simulink model "ulise_internal_v0"  (R2025b)
settings: Solver=FixedStepDiscrete  StartTime=0.0  StopTime=999  FixedStep=1  RelTol=1e-3
model workspace (MAT data in the model file):
  Something = 3
values from neighbouring files (symbols this model uses):
  A = [0.5    2   0   0   0 ... (first row only)    [simulink_ULISE.m]
  B = zeros(size(A,1),1)    [simulink_ULISE.m]
  C = blkdiag(1,1,1,1,1)    [simulink_ULISE.m]
  D = zeros(size(C,1),1)    [simulink_ULISE.m]
  G = [1  0   -0.3 ... (first row only)    [simulink_ULISE.m]
  H = [0  0   1 ... (first row only)    [simulink_ULISE.m]
  K = 1000    [simulink_ULISE.m]
  Q = 1e-4* [1    0   0   0   0 ... (first row only)    [simulink_ULISE.m]
  R = 1e-2* [1    0   0   0.5 0 ... (first row only)    [simulink_ULISE.m]
  x = zeros(size(A,1),K)    [simulink_ULISE.m]
  x0 = zeros(size(A,1),1)    [simulink_ULISE.m]
undefined symbols (not defined in the file or in its folder): P
libraries: dspinverses x1
settings Model: Creator=savan  LastModifiedBy=daniellawson

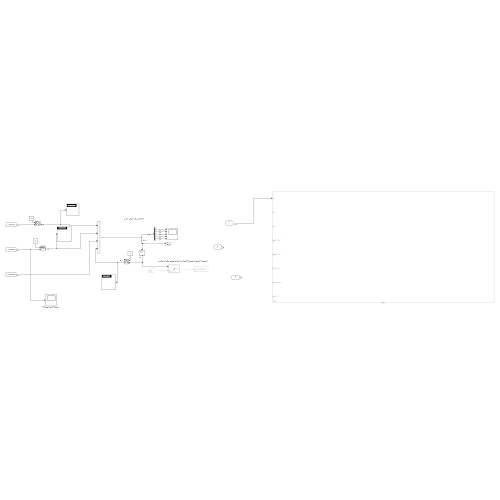
[thumbnail: Simulink's stored preview of the top-level diagram]
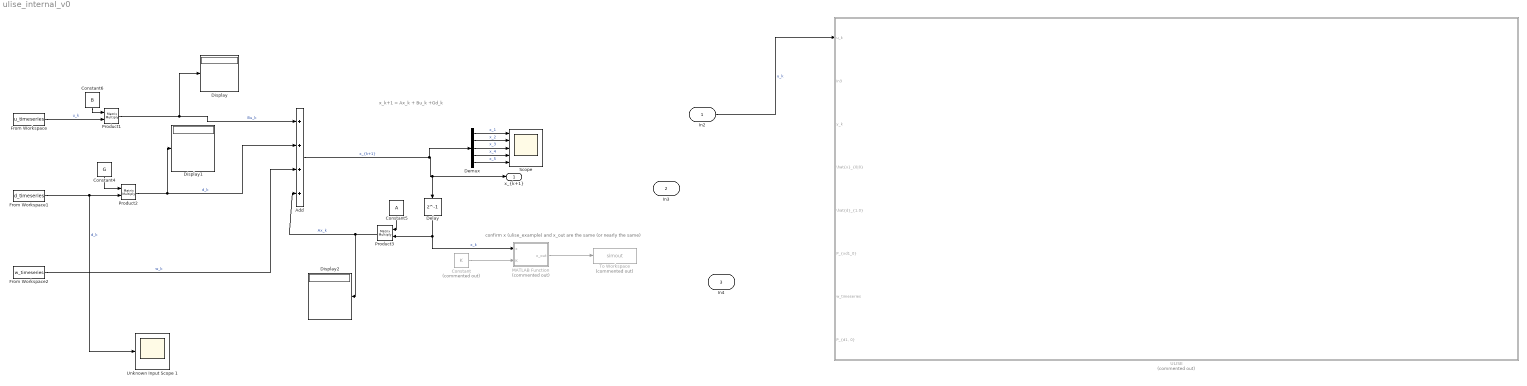
== system ulise_internal_v0 ==
  note: x_k+1 = Ax_k + Bu_k +Gd_k
  note: confirm x (ulise_example) and x_out are the same (or nearly the same)
  In2 : Inport
  In3 : Inport  Port=2
  In4 : Inport  Port=3
  Add : Sum  Inputs=++++
  Constant : Constant  Commented=on  Value=K
  Constant4 : Constant  Value=G
  Constant5 : Constant  Value=A
  Constant6 : Constant  Value=B
  Delay : Delay  DelayLength=1  InitialCondition=x0
  Demux : Demux  Outputs=size(x,1)
  Display : Display
  Display1 : Display
  Display2 : Display
  From Workspace : FromWorkspace  VariableName=u_timeseries
  From Workspace1 : FromWorkspace  VariableName=d_timeseries
  From Workspace2 : FromWorkspace  VariableName=w_timeseries
  MATLAB Function : MATLAB Function  Commented=on  TreatAsAtomicUnit=on
  Product1 : Product  Multiplication=Matrix(*)
  Product2 : Product  Multiplication=Matrix(*)
  Product3 : Product  Multiplication=Matrix(*)
  Scope : Scope  NumInputPorts=5
      settings: Title=ULISE States vs time  ActiveDisplayYMinimum=-16.811672647044393  ActiveDisplayYMaximum=16.458758069457645  YLabel=State x_1  DataLoggingVariableName=ScopeData4
  To Workspace : ToWorkspace  Commented=on  VariableName=simout  SaveFormat=Timeseries  SampleTime=-1
  ULISE : Subsystem  Commented=on
  Unknown Input Scope 1 : Scope
      settings: ActiveDisplayYMinimum=-6.4699830626674188  ActiveDisplayYMaximum=4.8185110652200844  DataLoggingVariableName=ScopeData2
  "x_{k+1}" : Outport
  wires:
  In2/1 -> ULISE/1(u_k)  "u_k"
  From Workspace2/1 -> Add/3  "w_k"
  Constant4/1 -> Product2/1
  Add/1 -> Demux/1, "x_{k+1}"/1, Delay/1  "x_{k+1}"
  From Workspace/1 -> Product1/2  "u_k"
  From Workspace1/1 -> Unknown Input Scope 1/1, Product2/2  "d_k"
  Delay/1 -> MATLAB Function/1(x), Product3/2  "x_k"
  Constant5/1 -> Product3/1
  Product3/1 -> Display2/1, Add/4  "Ax_k"
  Constant6/1 -> Product1/1
  Product1/1 -> Display/1, Add/1  "Bu_k"
  Demux/2 -> Scope/2  "x_2"
  Demux/5 -> Scope/5  "x_5"
  Demux/4 -> Scope/4  "x_4"
  Demux/3 -> Scope/3  "x_3"
  Demux/1 -> Scope/1  "x_1"
  Product2/1 -> Add/2, Display1/1  "d_k"
  Constant/1 -> MATLAB Function/2(K)
  MATLAB Function/1(x_out) -> To Workspace/1

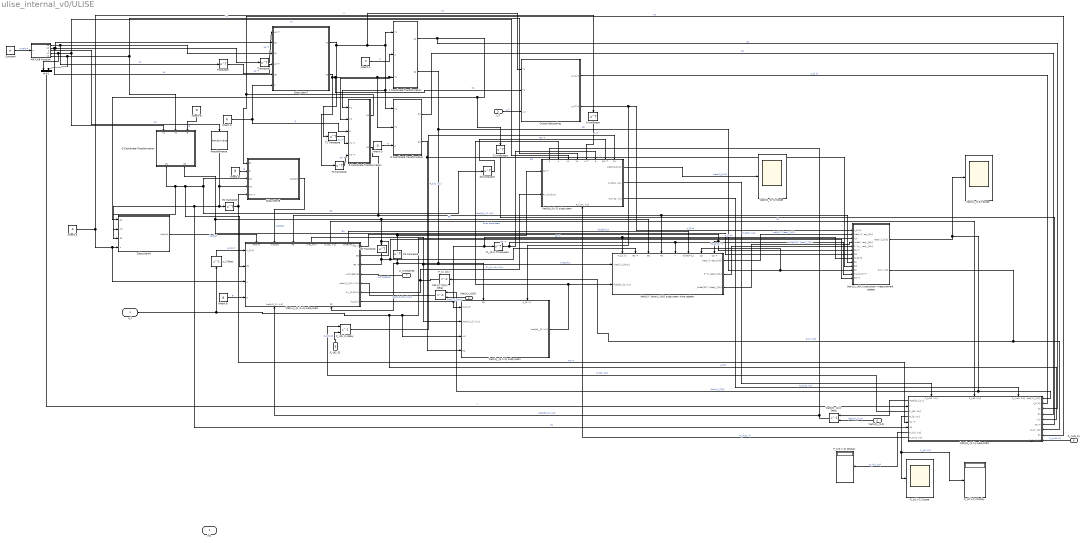
== system ulise_internal_v0/ULISE ==
  u_k : Inport
  In3 : Inport  Port=2
  y_k : Inport  Port=3
  "\\hat{x}_{0|0}" : Inport  Port=4
  "\\hat{d}_{1,0}" : Inport  Port=5
  "P_{xd1_0}" : Inport  Port=6
  w_timeseries : Inport  Port=7
  "P_{d1, 0}" : Inport  Port=8
  A transpose : Math  Operator=transpose
  C Coordinate Transformation : Subsystem
  C1 transpose : Math  Operator=transpose
  C2 transpose : Math  Operator=transpose
  Constant : Constant  Value=H
  D Coordinate Transformation : Subsystem
  G Coordinate Transformation : Subsystem
  G1 transpose : Math  Operator=transpose
  G2 Transpose : Math  Operator=transpose
  Inherit A : Constant  Value=A
  Inherit B : Constant  Value=B
  Inherit C : Constant  Value=C
  Inherit D : Constant  Value=D
  Inherit G : Constant  Value=G
  Inherit Q : Constant  Value=Q
  Inherit R : Constant  Value=R
  M1 transpose : Math  Operator=transpose
  MATLAB Function : MATLAB Function  TreatAsAtomicUnit=on
  "M_{2,k} Ttranspose" : Math  Operator=transpose
  Mux1 : Mux  Inputs=2
  Output Decoupling : Subsystem
  "P_{d, k-1} Display" : Display
  "P_{d, k-1} Scope" : Scope
      settings: DataLoggingVariableName=ScopeData3
  "P_{d1, k} Delay" : Delay  DelayLength=1  InitialConditionSource=Input port
      settings: InputPortMap=u0,p4
  "P_{x, k|k}" : Delay  DelayLength=1  InputProcessing=Columns as channels (frame based)
  "P_{xd, k-1} Display" : Display
  Pseudoinverse : dspinverses/Pseudoinverse  wanterr=off  SimulateUsing=Interpreted execution
  R Coordinate Transformation : Subsystem
  Subsystem6 : Subsystem
  Subsystem7 : Subsystem
  Subsystem8 : Subsystem
  "T1 Transpose " : Math  Operator=transpose
  T2 transpose : Math  Operator=transpose
  Transpose : Math  Operator=transpose
  Transpose1 : Math  Operator=transpose
  "\\hat{d}_{1, k} subsystem" : Subsystem
      settings: PortSchema="{\"entries\":[{\"content\":{\"sides\":[{\"content\":{\"connectorIds\":[\"Out1\",\"In1\",\"Out2\",\"Out3\",\"In2\",\"In3\",\"Out4\",\"Out5\"]},\"type\":\"ConnectorPlacement.EquallySpacedRectSide\",\"uuid\":\"a8af2826-9236-4219-ae2d-45ac01acad00\"},{\"content\":{\"connectorIds\":[\"In7\",\"In8\",\"In9\",\"In10\",\"In11\",\"In12\",\"In13\",\"In14\",\"In15\"],\"side\":\"RIGHT\"},\"type\":\"ConnectorPlacement.EquallySpacedRectSide\",\"uuid\":\"84eedaf4-945b-47e5-8cdc-84485c85dbd7\"},{\"content\":{\"connectorIds\":[\"In4\",\"In5\",\"In6\"],\"side\":\"TOP\"},\"type\":\"ConnectorPlacement.EquallySpacedRectSide\",\"uuid\":\"fbb834b4-c5e3-4ccc-9caa-e0274664c032\"}]},\"type\":\"ConnectorPlacement.EquallySpacedConnector\",\"uuid\":\"b7ff194e-a9c7-4e60-ae4f-2e8181f239f0\"}],\"packageUris\":[\"http://schema.mathworks.com/mf0/Connector/R2020b\"],\"version\":\"1.0\"}"
  "\\hat{d}_{1,k} Delay" : Delay  DelayLength=1  InitialConditionSource=Input port
      settings: InputPortMap=u0,p4
  "\\hat{d}_{2, k-1} subsystem" : Subsystem
      settings: PortSchema="{\"entries\":[{\"content\":{\"sides\":[{\"content\":{\"connectorIds\":[\"In1\",\"In2\",\"In3\",\"In4\"]},\"type\":\"ConnectorPlacement.EquallySpacedRectSide\",\"uuid\":\"5ac934c2-57a8-4f9d-b5fe-e946aa8ff042\"},{\"content\":{\"connectorIds\":[\"Out1\"],\"side\":\"RIGHT\"},\"type\":\"ConnectorPlacement.EquallySpacedRectSide\",\"uuid\":\"6cada4e5-46f2-404a-9388-706781b4a543\"},{\"content\":{\"connectorIds\":[\"In5\",\"In6\"],\"side\":\"TOP\"},\"type\":\"ConnectorPlacement.EquallySpacedRectSide\",\"uuid\":\"17126271-5fec-450a-b828-57096aea8cbe\"}]},\"type\":\"ConnectorPlacement.EquallySpacedConnector\",\"uuid\":\"bc02aed0-427b-4e3d-8c25-36b44785aefd\"}],\"packageUris\":[\"http://schema.mathworks.com/mf0/Connector/R2020b\"],\"version\":\"1.0\"}"
  "\\hat{d}_{k-1} Scope" : Scope
  "\\hat{d}_{k-1} subsystem" : Subsystem
      settings: PortSchema="{\"entries\":[{\"content\":{\"sides\":[{\"content\":{\"connectorIds\":[\"In1\",\"In2\"]},\"type\":\"ConnectorPlacement.EquallySpacedRectSide\",\"uuid\":\"b345720d-76db-4e73-980e-036df274b869\"},{\"content\":{\"connectorIds\":[\"Out1\",\"Out2\",\"Out3\"],\"side\":\"RIGHT\"},\"type\":\"ConnectorPlacement.EquallySpacedRectSide\",\"uuid\":\"83530859-5e45-4fdc-8627-b960bf21f0f3\"},{\"content\":{\"connectorIds\":[\"In3\",\"In4\",\"In5\",\"In6\",\"In7\",\"In8\",\"In9\",\"In10\"],\"side\":\"TOP\"},\"type\":\"ConnectorPlacement.EquallySpacedRectSide\",\"uuid\":\"a90177c3-54b6-4f29-9d5b-286734427aaf\"},{\"content\":{\"connectorIds\":[\"In11\"],\"side\":\"BOTTOM\"},\"type\":\"ConnectorPlacement.EquallySpacedRectSide\",\"uuid\":\"f56d1d5c-dc27-4a78-b936-b8320e40f46c\"}]},\"type\":\"ConnectorPlacement.EquallySpacedConnector\",\"uuid\":\"37499251-74e7-4e57-895e-3c0e103ac17a\"}],\"packageUris\":[\"http://schema.mathworks.com/mf0/Connector/R2020b\"],\"version\":\"1.0\"}"
  "\\hat{x}^{star}_{k|k} subsystem: time update" : Subsystem
      settings: PortSchema="{\"entries\":[{\"content\":{\"sides\":[{\"content\":{\"connectorIds\":[\"In1\",\"In2\"]},\"type\":\"ConnectorPlacement.EquallySpacedRectSide\",\"uuid\":\"5830eee7-c567-4dea-997c-8a153f47a1e5\"},{\"content\":{\"connectorIds\":[\"Out1\",\"Out2\",\"Out3\"],\"side\":\"RIGHT\"},\"type\":\"ConnectorPlacement.EquallySpacedRectSide\",\"uuid\":\"fc2d532a-0741-4542-9657-5f6e7d81890d\"},{\"content\":{\"connectorIds\":[\"In3\",\"In4\",\"In5\",\"In6\",\"In7\",\"In8\",\"In9\",\"In10\"],\"side\":\"TOP\"},\"type\":\"ConnectorPlacement.EquallySpacedRectSide\",\"uuid\":\"665916ba-7ee7-4559-9e7e-f21672fe0f8a\"}]},\"type\":\"ConnectorPlacement.EquallySpacedConnector\",\"uuid\":\"6ca8778a-6b89-47d3-9c62-becd7cf79fd9\"}],\"packageUris\":[\"http://schema.mathworks.com/mf0/Connector/R2020b\"],\"version\":\"1.0\"}"
  "\\hat{x}_{k | k-1} subsystem" : Subsystem
      settings: PortSchema="{\"entries\":[{\"content\":{\"sides\":[{\"content\":{\"connectorIds\":[\"In1\",\"In2\",\"In3\",\"In4\"]},\"type\":\"ConnectorPlacement.EquallySpacedRectSide\",\"uuid\":\"a8af2826-9236-4219-ae2d-45ac01acad00\"},{\"content\":{\"connectorIds\":[\"In10\",\"In11\",\"In12\",\"In13\",\"In14\",\"In15\",\"Out1\"],\"side\":\"RIGHT\"},\"type\":\"ConnectorPlacement.EquallySpacedRectSide\",\"uuid\":\"84eedaf4-945b-47e5-8cdc-84485c85dbd7\"},{\"content\":{\"connectorIds\":[\"In5\",\"In6\",\"In7\",\"Out2\",\"Out3\",\"Out4\"],\"side\":\"TOP\"},\"type\":\"ConnectorPlacement.EquallySpacedRectSide\",\"uuid\":\"fbb834b4-c5e3-4ccc-9caa-e0274664c032\"},{\"content\":{\"connectorIds\":[\"In8\",\"In9\"],\"side\":\"BOTTOM\"},\"type\":\"ConnectorPlacement.EquallySpacedRectSide\",\"uuid\":\"4274c574-9492-4236-af77-13af9c9f0a33\"}]},\"type\":\"ConnectorPlacement.EquallySpacedConnector\",\"uuid\":\"b7ff194e-a9c7-4e60-ae4f-2e8181f239f0\"}],\"packageUris\":[\"http://schema.mathworks.com/mf0/Connector/R2020b\"],\"version\":\"1.0\"}"
  "\\hat{x}_{k|k} Delay" : Delay  DelayLength=1  InitialConditionSource=Input port
      settings: InputPortMap=u0,p4
  "\\hat{x}_{k|k} Scope" : Scope
  "\\hat{x}_{k|k} subsystem: measurement update" : Subsystem
  u_k Delay : Delay  DelayLength=1  InputProcessing=Columns as channels (frame based)
  wires:
  "\\hat{d}_{k-1} subsystem"/1("\\hat{d}_{k-1}") -> "\\hat{d}_{k-1} Scope"/1  "\\hat{d}_{k-1}"
  u_k Delay/1 -> "\\hat{x}_{k | k-1} subsystem"/1("u_{k-1}")  "u_{k-1}"
  u_k/1 -> "\\hat{d}_{1, k} subsystem"/11(u_k), "\\hat{d}_{2, k-1} subsystem"/3(u_k), "\\hat{x}_{k|k} subsystem: measurement update"/3(u_k), u_k Delay/1  "u_{k}"
  "\\hat{x}^{star}_{k|k} subsystem: time update"/1("\\hat{x}^star_{k|k}") -> "\\hat{x}_{k|k} subsystem: measurement update"/2("\\hat{x}^star_{k|k}")  "\\hat{x}^{star}_{k|k}"
  "\\hat{d}_{1, k} subsystem"/1("\\hat{d}_{1,k}") -> "\\hat{d}_{1,k} Delay"/1
  "\\hat{x}_{k | k-1} subsystem"/2(xhat_k|k-1) -> "\\hat{d}_{2, k-1} subsystem"/2("\\hat{x}_{k | k-1}"), "\\hat{x}^{star}_{k|k} subsystem: time update"/1("\\hat{x}_{k|k-1}")  "xhat_k|k-1"
  "\\hat{x}_{k|k} subsystem: measurement update"/1("\\hat{x}_{k|k}") -> "\\hat{x}_{k|k} Scope"/1, "\\hat{x}_{k|k} Delay"/1, "\\hat{d}_{1, k} subsystem"/7("\\hat{x}_{k|k}")  "\\hat{x}_{k|k}"
  "\\hat{d}_{2, k-1} subsystem"/1("\\hat{d}_{2, k-1}") -> "\\hat{d}_{k-1} subsystem"/4("\\hat{d}_{2, k-1}"), "\\hat{x}^{star}_{k|k} subsystem: time update"/2("\\hat{d}_{2, k-1}")  "\\hat{d}_{2, k-1}"
  Constant/1 -> MATLAB Function/1(H)  "Inherit H"
  MATLAB Function/1(U1) -> Subsystem7/3(U1), Transpose/1  "U1"
  MATLAB Function/2(U2) -> Subsystem7/2(U2), Transpose1/1, Subsystem7/5(U3)  "U2"
  Inherit R/1 -> Subsystem7/6(R), R Coordinate Transformation/3(R)  "R"
  MATLAB Function/3(S) -> Pseudoinverse/1  "M1"
  Inherit A/1 -> "\\hat{x}_{k | k-1} subsystem"/3(A), Subsystem6/4(A), A transpose/1  "A"
  Subsystem6/1("\\hat{A}") -> "\\hat{x}_{k | k-1} subsystem"/5("\\hat{A}")  "\\hat{A}"
  Subsystem7/2(T2) -> Output Decoupling/2(T2), R Coordinate Transformation/2(T2), C Coordinate Transformation/3(T2), D Coordinate Transformation/2(T2), T2 transpose/1  "T2"
  Subsystem7/1(T1) -> Output Decoupling/1(T1), D Coordinate Transformation/1(T1), R Coordinate Transformation/1(T1), C Coordinate Transformation/1(T1), "T1 Transpose "/1  "T1"
  Transpose1/1 -> Subsystem7/1(U2^T)  "U2^T"
  Transpose/1 -> Subsystem7/4(U1^T)  "U1^T"
  Pseudoinverse/1 -> M1 transpose/1, "\\hat{d}_{1, k} subsystem"/3(M1), Subsystem6/2(M1), Subsystem8/4(M1)  "M1"
  MATLAB Function/4(V1) -> Mux1/1, G Coordinate Transformation/1(V1), "\\hat{d}_{k-1} subsystem"/5(V1)  "V1"
  MATLAB Function/5(V2) -> Mux1/2, "\\hat{d}_{k-1} subsystem"/6(V2), G Coordinate Transformation/2(V2)  "V2"
  Inherit G/1 -> G Coordinate Transformation/3(G)  "G"
  C2 transpose/1 -> "\\hat{x}^{star}_{k|k} subsystem: time update"/10(C2^T), "\\hat{x}_{k|k} subsystem: measurement update"/6(C2^T), "\\hat{x}_{k | k-1} subsystem"/10(C2^T), "\\hat{d}_{k-1} subsystem"/1(C2^T)  "C2^T"
  G Coordinate Transformation/1(G1) -> Subsystem6/3(G1), "\\hat{x}_{k | k-1} subsystem"/2(G1), Subsystem8/3(G1), G1 transpose/1  "G1"
  Inherit Q/1 -> Subsystem8/2(Q)  "Q"
  M1 transpose/1 -> "\\hat{d}_{1, k} subsystem"/2(M1^T), Subsystem8/5(M1^T)  "M1^T"
  Subsystem8/1("\\hat{Q}") -> "\\hat{x}_{k | k-1} subsystem"/6("\\hat{Q}")  "\\hat{Q}"
  "T1 Transpose "/1 -> R Coordinate Transformation/4(T1^T)  "T1^T"
  T2 transpose/1 -> R Coordinate Transformation/5(T2^T)  "T2^T"
  R Coordinate Transformation/1(R1) -> Subsystem8/1(R1), "\\hat{d}_{1, k} subsystem"/14(R1)  "R1"
  R Coordinate Transformation/2(R2) -> "\\hat{x}^{star}_{k|k} subsystem: time update"/6(R2), "\\hat{x}_{k|k} subsystem: measurement update"/9(R2), "\\hat{x}_{k | k-1} subsystem"/7(R2)  "R2"
  Inherit D/1 -> D Coordinate Transformation/3(D)  "D"
  C Coordinate Transformation/2(C2) -> "\\hat{x}_{k|k} subsystem: measurement update"/11(C2), "\\hat{x}^{star}_{k|k} subsystem: time update"/9(C2), "\\hat{d}_{2, k-1} subsystem"/5(C2), C2 transpose/1, "\\hat{x}_{k | k-1} subsystem"/9(C2)  "C2"
  Inherit C/1 -> C Coordinate Transformation/2(C)  "C"
  G Coordinate Transformation/2(G2) -> "\\hat{x}_{k|k} subsystem: measurement update"/7(G2), "\\hat{x}^{star}_{k|k} subsystem: time update"/5(G2), G2 Transpose/1, "\\hat{x}_{k | k-1} subsystem"/11(G2)  "G2"
  G2 Transpose/1 -> "\\hat{x}_{k | k-1} subsystem"/12(G2^T), "\\hat{x}^{star}_{k|k} subsystem: time update"/4(G2^T), "\\hat{x}_{k|k} subsystem: measurement update"/13(G2^T)  "G2^T"
  Inherit B/1 -> "\\hat{x}_{k | k-1} subsystem"/4(B)  "B"
  "\\hat{x}_{k | k-1} subsystem"/1("M_{2,k}") -> "\\hat{d}_{2, k-1} subsystem"/1("M_{2,k}"), "\\hat{x}^{star}_{k|k} subsystem: time update"/3("M_{2, k}"), "\\hat{x}_{k|k} subsystem: measurement update"/8("M_{2,k}"), "M_{2,k} Ttranspose"/1  "M_{2,k}"
  y_k/1 -> Output Decoupling/3(y_k)  "y_k"
  "P_{x, k|k}"/1 -> "\\hat{x}_{k | k-1} subsystem"/15("Px_{k-1|k-1}"), "\\hat{d}_{k-1} subsystem"/2("Px_{k-1|k-1}")  "Px_{x, k-1 | k-1}"
  "\\hat{x}_{k|k} subsystem: measurement update"/2("P_{x, k|k}") -> "\\hat{d}_{1, k} subsystem"/13("P_{x, k|k}"), "P_{x, k|k}"/1  "P_{x, k|k}"
  D Coordinate Transformation/2(D2) -> "\\hat{x}_{k|k} subsystem: measurement update"/10(D2), "\\hat{d}_{2, k-1} subsystem"/4(D2)  "D2"
  "\\hat{d}_{1,k} Delay"/1 -> "\\hat{d}_{k-1} subsystem"/3("\\hat{d}_{1, k-1}"), "\\hat{x}_{k | k-1} subsystem"/8("\\hat{d}_{1, k-1}")  "\\hat{d}_{1, k-1}"
  A transpose/1 -> "\\hat{d}_{k-1} subsystem"/7(A^T)  "A^T"
  C1 transpose/1 -> "\\hat{d}_{1, k} subsystem"/12(C1^T)  "C1"
  G1 transpose/1 -> "\\hat{d}_{k-1} subsystem"/9(G1^T)  "G1^T"
  "M_{2,k} Ttranspose"/1 -> "\\hat{x}^{star}_{k|k} subsystem: time update"/7("(M_{2, k})^T"), "\\hat{x}_{k|k} subsystem: measurement update"/12("(M_{2,k})^T"), "\\hat{d}_{k-1} subsystem"/8("(M_{2,k})^T")  "(M_{2,k})^T"
  Output Decoupling/2("z_{2,k}") -> "\\hat{x}_{k|k} subsystem: measurement update"/1("z_{2,k}"), "\\hat{d}_{2, k-1} subsystem"/6("z_{2, k}")  "z_{2,k}"
  "\\hat{x}^{star}_{k|k} subsystem: time update"/3("\\tilde{R2}^{star}_{k|k}") -> "\\hat{x}_{k|k} subsystem: measurement update"/4("\\tilde{R2}^{star}_{k|k}")  "\\tilde{R2}^{star}_{k|k}"
  "\\hat{x}^{star}_{k|k} subsystem: time update"/2("P^{x_star}_{k|k}") -> "\\hat{x}_{k|k} subsystem: measurement update"/5("P^{x_star}_{k|k}")
  Mux1/1 -> "\\hat{d}_{1, k} subsystem"/1(V)  "V"
  "\\hat{d}_{k-1} subsystem"/2("P_{d12, k-1}") -> "\\hat{d}_{1, k} subsystem"/4("P_{d12, k-1}")  "P_{d12, k-1}"
  "\\hat{d}_{k-1} subsystem"/3("P_{xd2, k-1}") -> "\\hat{d}_{1, k} subsystem"/6("P_{xd2, k-1}")  "P_{xd2, k-1}"
  "\\hat{x}_{k | k-1} subsystem"/3("P_{d2, k-1}") -> "\\hat{d}_{1, k} subsystem"/5("P_{d2, k-1}")  "priori subsystem"
  Output Decoupling/1("z_{1,k}") -> "\\hat{d}_{1, k} subsystem"/8("z_{1,k}")  "z_{1,k}"
  "\\hat{x}_{k|k} Delay"/1 -> "\\hat{x}_{k | k-1} subsystem"/14("\\hat{x}_{k-1 | k-1}")  "\\hat{x}_{k-1 | k-1}"
  "\\hat{x}_{0|0}"/1 -> "\\hat{x}_{k|k} Delay"/2  "\\hat{x}_{0|0}"
  "\\hat{d}_{1,0}"/1 -> "\\hat{d}_{1,k} Delay"/2  "\\hat{d}_{1,0}"
  C Coordinate Transformation/1(C1) -> "\\hat{d}_{1, k} subsystem"/9(C1), C1 transpose/1, Subsystem6/1(C1)  "C1"
  "P_{xd1_0}"/1 -> "\\hat{d}_{1, k} subsystem"/15("P_{xd1, 0}")  "P_{xd1, 0}"
  D Coordinate Transformation/1(D1) -> "\\hat{d}_{1, k} subsystem"/10(D1)  "D1"
  w_timeseries/1 -> "\\hat{x}_{k | k-1} subsystem"/13(w_timeseries)  "w_timeseries"
  "\\hat{d}_{1, k} subsystem"/4("P_{xd, k-1}") -> "P_{xd, k-1} Display"/1  "P_{xd, k-1}"
  "\\hat{d}_{1, k} subsystem"/2("P_{d1, k|k}") -> "P_{d1, k} Delay"/1  "P_{d1, k|k}"
  "P_{d1, 0}"/1 -> "P_{d1, k} Delay"/2  "P_{d1,0}"
  "P_{d1, k} Delay"/1 -> "\\hat{d}_{k-1} subsystem"/10("P_{d1, k-1}")  "P_{d1, k-1}"
  "\\hat{d}_{1, k} subsystem"/5("P_{xd1, k-1}") -> "\\hat{d}_{k-1} subsystem"/11("P_{xd1, k-1}")  "P_{xd1, k}"
  "\\hat{d}_{1, k} subsystem"/3("P_{d, k-1}") -> "P_{d, k-1} Display"/1, "P_{d, k-1} Scope"/1  "P_{d, k-1}"
  "\\hat{x}_{k | k-1} subsystem"/4("\\tilde{P}_k") -> "\\hat{x}^{star}_{k|k} subsystem: time update"/8("\\tilde{P}_k")  "\\tilde{P}_k"

== system ulise_internal_v0/ULISE/C Coordinate Transformation ==
  T1 : Inport
  C : Inport  Port=2
  T2 : Inport  Port=3
  Matrix Multiply2 : Product  Multiplication=Matrix(*)
  Matrix Multiply3 : Product  Multiplication=Matrix(*)
  C1 : Outport
  C2 : Outport  Port=2
  wires:
  Matrix Multiply2/1 -> C2/1  "C2"
  T2/1 -> Matrix Multiply2/1  "T2"
  Matrix Multiply3/1 -> C1/1  "C1"
  T1/1 -> Matrix Multiply3/1  "T1"
  C/1 -> Matrix Multiply3/2, Matrix Multiply2/2  "C"

== system ulise_internal_v0/ULISE/D Coordinate Transformation ==
  T1 : Inport
  T2 : Inport  Port=2
  D : Inport  Port=3
  Matrix Multiply4 : Product  Multiplication=Matrix(*)
  Matrix Multiply5 : Product  Multiplication=Matrix(*)
  D1 : Outport
  D2 : Outport  Port=2
  wires:
  T2/1 -> Matrix Multiply5/1  "T2"
  Matrix Multiply4/1 -> D1/1  "D1"
  T1/1 -> Matrix Multiply4/1  "T1"
  Matrix Multiply5/1 -> D2/1  "D2"
  D/1 -> Matrix Multiply4/2, Matrix Multiply5/2  "D"

== system ulise_internal_v0/ULISE/G Coordinate Transformation ==
  V1 : Inport
  V2 : Inport  Port=2
  G : Inport  Port=3
  Matrix Multiply6 : Product  Multiplication=Matrix(*)
  Matrix Multiply7 : Product  Multiplication=Matrix(*)
  G1 : Outport
  G2 : Outport  Port=2
  wires:
  Matrix Multiply6/1 -> G1/1  "G1"
  Matrix Multiply7/1 -> G2/1  "G2"
  V2/1 -> Matrix Multiply7/2  "V2"
  V1/1 -> Matrix Multiply6/2  "V1"
  G/1 -> Matrix Multiply6/1, Matrix Multiply7/1  "G"

== system ulise_internal_v0/ULISE/Output Decoupling ==
  T1 : Inport
  T2 : Inport  Port=2
  y_k : Inport  Port=3
  Matrix Multiply1 : Product  Multiplication=Matrix(*)
  Matrix Multiply2 : Product  Multiplication=Matrix(*)
  "z_{1,k}" : Outport
  "z_{2,k}" : Outport  Port=2
  wires:
  T2/1 -> Matrix Multiply2/1
  Matrix Multiply1/1 -> "z_{1,k}"/1  "z_{1,k}"
  Matrix Multiply2/1 -> "z_{2,k}"/1  "z_{2,k}"
  T1/1 -> Matrix Multiply1/1
  y_k/1 -> Matrix Multiply2/2, Matrix Multiply1/2

== system ulise_internal_v0/ULISE/R Coordinate Transformation ==
  T1 : Inport
  T2 : Inport  Port=2
  R : Inport  Port=3
  T1^T : Inport  Port=4
  T2^T : Inport  Port=5
  Matrix Multiply1 : Product  Inputs=3  Multiplication=Matrix(*)
  Matrix Multiply8 : Product  Inputs=3  Multiplication=Matrix(*)
  R1 : Outport
  R2 : Outport  Port=2
  wires:
  T2^T/1 -> Matrix Multiply8/3  "T2^T"
  T2/1 -> Matrix Multiply8/1  "T2"
  T1/1 -> Matrix Multiply1/1  "T1"
  Matrix Multiply1/1 -> R1/1  "R1"
  T1^T/1 -> Matrix Multiply1/3  "T1^T"
  Matrix Multiply8/1 -> R2/1  "R2"
  R/1 -> Matrix Multiply8/2, Matrix Multiply1/2  "R"

== system ulise_internal_v0/ULISE/Subsystem6 ==
  C1 : Inport
  M1 : Inport  Port=2
  G1 : Inport  Port=3
  A : Inport  Port=4
  Add1 : Sum
  Matrix Multiply8 : Product  Inputs=3  Multiplication=Matrix(*)
  "\\hat{A}" : Outport
  wires:
  C1/1 -> Matrix Multiply8/3
  M1/1 -> Matrix Multiply8/2
  Add1/1 -> "\\hat{A}"/1  "\\hat{A}"
  A/1 -> Add1/1
  G1/1 -> Matrix Multiply8/1
  Matrix Multiply8/1 -> Add1/2

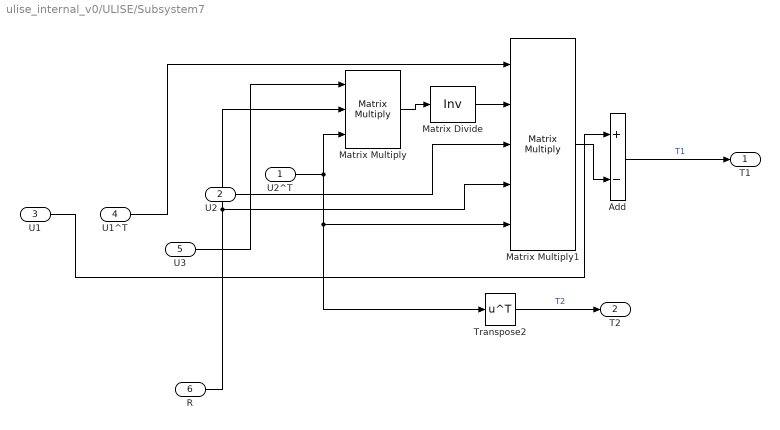
== system ulise_internal_v0/ULISE/Subsystem7 ==
  U2^T : Inport
  U2 : Inport  Port=2
  U1 : Inport  Port=3
  U1^T : Inport  Port=4
  U3 : Inport  Port=5
  R : Inport  Port=6
  Add : Sum  Inputs=+-
  Matrix Divide : Product  Inputs=/  Multiplication=Matrix(*)
  Matrix Multiply : Product  Inputs=3  Multiplication=Matrix(*)
  Matrix Multiply1 : Product  Inputs=5  Multiplication=Matrix(*)
  Transpose2 : Math  Operator=transpose
  T1 : Outport
  T2 : Outport  Port=2
  wires:
  Transpose2/1 -> T2/1  "T2"
  U1^T/1 -> Matrix Multiply1/1
  Add/1 -> T1/1  "T1"
  Matrix Divide/1 -> Matrix Multiply1/2
  Matrix Multiply/1 -> Matrix Divide/1
  U1/1 -> Add/1
  R/1 -> Matrix Multiply/2, Matrix Multiply1/4
  U2/1 -> Matrix Multiply1/3
  U3/1 -> Matrix Multiply/1
  Matrix Multiply1/1 -> Add/2
  U2^T/1 -> Matrix Multiply/3, Transpose2/1, Matrix Multiply1/5

== system ulise_internal_v0/ULISE/Subsystem8 ==
  R1 : Inport
  Q : Inport  Port=2
  G1 : Inport  Port=3
  M1 : Inport  Port=4
  M1^T : Inport  Port=5
  Add : Sum
  Matrix Multiply : Product  Inputs=4  Multiplication=Matrix(*)
  "\\hat{Q}" : Outport
  wires:
  Q/1 -> Add/1
  R1/1 -> Matrix Multiply/3
  M1^T/1 -> Matrix Multiply/4
  G1/1 -> Matrix Multiply/1
  Add/1 -> "\\hat{Q}"/1  "\\hat{Q}"
  M1/1 -> Matrix Multiply/2
  Matrix Multiply/1 -> Add/2

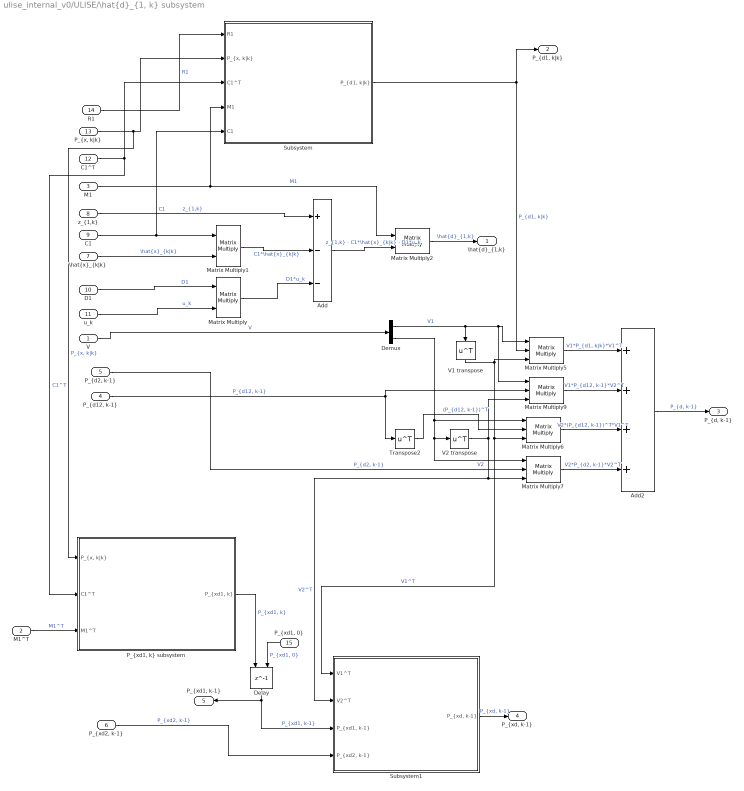
== system ulise_internal_v0/ULISE/\hat{d}_{1, k} subsystem ==
  V : Inport
  M1^T : Inport  Port=2
  M1 : Inport  Port=3
  "P_{d12, k-1}" : Inport  Port=4
  "P_{d2, k-1}" : Inport  Port=5
  "P_{xd2, k-1}" : Inport  Port=6
  "\\hat{x}_{k|k}" : Inport  Port=7
  "z_{1,k}" : Inport  Port=8
  C1 : Inport  Port=9
  D1 : Inport  Port=10
  u_k : Inport  Port=11
  C1^T : Inport  Port=12
  "P_{x, k|k}" : Inport  Port=13
  R1 : Inport  Port=14
  "P_{xd1, 0}" : Inport  Port=15
  Add : Sum  Inputs=+--
  Add2 : Sum  Inputs=++++
  Delay : Delay  DelayLength=1  InitialConditionSource=Input port  InitialCondition=P
      settings: InputPortMap=u0,p4
  Demux : Demux  Outputs=2
  Matrix Multiply : Product  Multiplication=Matrix(*)
  Matrix Multiply1 : Product  Multiplication=Matrix(*)
  Matrix Multiply2 : Product  Multiplication=Matrix(*)
  Matrix Multiply{5..7,9} (4 alike) : Product  Inputs=3  Multiplication=Matrix(*)
  "P_{xd1, k} subsystem" : Subsystem
  Subsystem : Subsystem
  Subsystem1 : Subsystem
  Transpose2 : Math  Operator=transpose
  V1 transpose : Math  Operator=transpose
  V2 transpose : Math  Operator=transpose
  "\\hat{d}_{1,k}" : Outport
  "P_{d1, k|k}" : Outport  Port=2
  "P_{d, k-1}" : Outport  Port=3
  "P_{xd, k-1}" : Outport  Port=4
  "P_{xd1, k-1}" : Outport  Port=5
  wires:
  "z_{1,k}"/1 -> Add/1  "z_{1,k}"
  M1/1 -> Matrix Multiply2/1, Subsystem/4(M1)  "M1"
  D1/1 -> Matrix Multiply/1  "D1"
  u_k/1 -> Matrix Multiply/2  "u_k"
  "\\hat{x}_{k|k}"/1 -> Matrix Multiply1/2  "\\hat{x}_{k|k}"
  C1/1 -> Subsystem/5(C1), Matrix Multiply1/1  "C1"
  Matrix Multiply/1 -> Add/3  "D1*u_k"
  Matrix Multiply1/1 -> Add/2  "C1*\\hat{x}_{k|k}"
  Add/1 -> Matrix Multiply2/2  "z_{1,k} - C1*\\hat{x}_{k|k} - D1*u_k"
  Matrix Multiply2/1 -> "\\hat{d}_{1,k}"/1  "\\hat{d}_{1,k}"
  "P_{x, k|k}"/1 -> Subsystem/2("P_{x, k|k}"), "P_{xd1, k} subsystem"/1("P_{x, k|k}")  "P_{x, k|k}"
  M1^T/1 -> "P_{xd1, k} subsystem"/3(M1^T)  "M1^T"
  C1^T/1 -> Subsystem/3(C1^T), "P_{xd1, k} subsystem"/2(C1^T)  "C1^T"
  "P_{xd1, k} subsystem"/1("P_{xd1, k}") -> Delay/1  "P_{xd1, k}"
  V/1 -> Demux/1  "V"
  Demux/1 -> Matrix Multiply9/1, Matrix Multiply5/1, V1 transpose/1  "V1"
  Demux/2 -> Matrix Multiply6/1, Matrix Multiply7/1, V2 transpose/1  "V2"
  V1 transpose/1 -> Subsystem1/1(V1^T), Matrix Multiply6/3, Matrix Multiply5/3  "V1^T"
  V2 transpose/1 -> Matrix Multiply9/3, Subsystem1/2(V2^T), Matrix Multiply7/3  "V2^T"
  Matrix Multiply7/1 -> Add2/4  "V2*P_{d2, k-1}*V2^T"
  Matrix Multiply6/1 -> Add2/3  "V2*(P_{d12, k-1})^T*V1^T"
  Matrix Multiply9/1 -> Add2/2  "V1*P_{d12, k-1}*V2^T"
  Matrix Multiply5/1 -> Add2/1  "V1*P_{d1, k|k}*V1^T"
  Add2/1 -> "P_{d, k-1}"/1  "P_{d, k-1}"
  "P_{d12, k-1}"/1 -> Transpose2/1, Matrix Multiply9/2  "P_{d12, k-1}"
  "P_{d2, k-1}"/1 -> Matrix Multiply7/2  "P_{d2, k-1}"
  Transpose2/1 -> Matrix Multiply6/2  "(P_{d12, k-1})^T"
  "P_{xd2, k-1}"/1 -> Subsystem1/4("P_{xd2, k-1}")  "P_{xd2, k-1}"
  Subsystem1/1("P_{xd, k-1}") -> "P_{xd, k-1}"/1  "P_{xd, k-1}"
  Delay/1 -> "P_{xd1, k-1}"/1, Subsystem1/3("P_{xd1, k-1}")  "P_{xd1, k-1}"
  "P_{xd1, 0}"/1 -> Delay/2  "P_{xd1, 0}"
  Subsystem/1("P_{d1, k|k}") -> "P_{d1, k|k}"/1, Matrix Multiply5/2  "P_{d1, k|k}"
  R1/1 -> Subsystem/1(R1)  "R1"

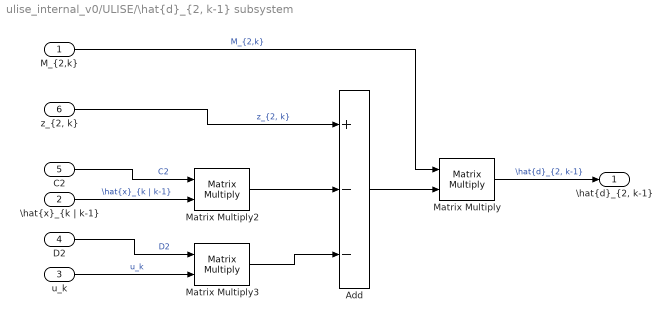
== system ulise_internal_v0/ULISE/\hat{d}_{2, k-1} subsystem ==
  "M_{2,k}" : Inport
  "\\hat{x}_{k | k-1}" : Inport  Port=2
  u_k : Inport  Port=3
  D2 : Inport  Port=4
  C2 : Inport  Port=5
  "z_{2, k}" : Inport  Port=6
  Add : Sum  Inputs=+--
  Matrix Multiply : Product  Multiplication=Matrix(*)
  Matrix Multiply2 : Product  Multiplication=Matrix(*)
  Matrix Multiply3 : Product  Multiplication=Matrix(*)
  "\\hat{d}_{2, k-1}" : Outport
  wires:
  "\\hat{x}_{k | k-1}"/1 -> Matrix Multiply2/2  "\\hat{x}_{k | k-1}"
  u_k/1 -> Matrix Multiply3/2  "u_k"
  D2/1 -> Matrix Multiply3/1  "D2"
  C2/1 -> Matrix Multiply2/1  "C2"
  "z_{2, k}"/1 -> Add/1  "z_{2, k}"
  "M_{2,k}"/1 -> Matrix Multiply/1  "M_{2,k}"
  Matrix Multiply2/1 -> Add/2
  Matrix Multiply3/1 -> Add/3
  Add/1 -> Matrix Multiply/2
  Matrix Multiply/1 -> "\\hat{d}_{2, k-1}"/1  "\\hat{d}_{2, k-1}"

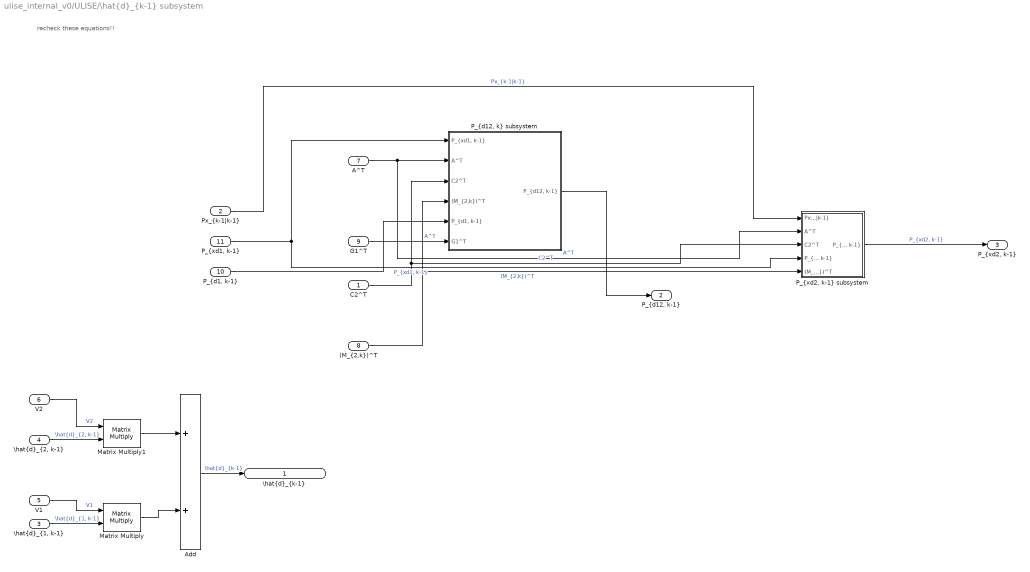
== system ulise_internal_v0/ULISE/\hat{d}_{k-1} subsystem ==
  note: recheck these equations!!
  C2^T : Inport
  "Px_{k-1|k-1}" : Inport  Port=2
  "\\hat{d}_{1, k-1}" : Inport  Port=3
  "\\hat{d}_{2, k-1}" : Inport  Port=4
  V1 : Inport  Port=5
  V2 : Inport  Port=6
  A^T : Inport  Port=7
  "(M_{2,k})^T" : Inport  Port=8
  G1^T : Inport  Port=9
  "P_{d1, k-1}" : Inport  Port=10
  "P_{xd1, k-1}" : Inport  Port=11
  Add : Sum
  Matrix Multiply : Product  Multiplication=Matrix(*)
  Matrix Multiply1 : Product  Multiplication=Matrix(*)
  "P_{d12, k} subsystem" : Subsystem
  "P_{xd2, k-1} subsystem" : Subsystem
  "\\hat{d}_{k-1}" : Outport
  "P_{d12, k-1}" : Outport  Port=2
  "P_{xd2, k-1}" : Outport  Port=3
  wires:
  "\\hat{d}_{1, k-1}"/1 -> Matrix Multiply/2  "\\hat{d}_{1, k-1}"
  V1/1 -> Matrix Multiply/1  "V1"
  "\\hat{d}_{2, k-1}"/1 -> Matrix Multiply1/2  "\\hat{d}_{2, k-1}"
  V2/1 -> Matrix Multiply1/1  "V2"
  Matrix Multiply/1 -> Add/2
  Matrix Multiply1/1 -> Add/1
  Add/1 -> "\\hat{d}_{k-1}"/1  "\\hat{d}_{k-1}"
  A^T/1 -> "P_{xd2, k-1} subsystem"/2(A^T), "P_{d12, k} subsystem"/2(A^T)  "A^T"
  C2^T/1 -> "P_{d12, k} subsystem"/3(C2^T), "P_{xd2, k-1} subsystem"/3(C2^T)  "C2^T"
  "(M_{2,k})^T"/1 -> "P_{d12, k} subsystem"/4("(M_{2,k})^T"), "P_{xd2, k-1} subsystem"/5("(M_{2,k})^T")  "(M_{2,k})^T"
  "Px_{k-1|k-1}"/1 -> "P_{xd2, k-1} subsystem"/1("Px_{k-1|k-1}")  "Px_{k-1|k-1}"
  "P_{d12, k} subsystem"/1("P_{d12, k-1}") -> "P_{d12, k-1}"/1
  G1^T/1 -> "P_{d12, k} subsystem"/6(G1^T)  "A^T"
  "P_{xd2, k-1} subsystem"/1("P_{xd2, k-1}") -> "P_{xd2, k-1}"/1  "P_{xd2, k-1}"
  "P_{d1, k-1}"/1 -> "P_{d12, k} subsystem"/5("P_{d1, k-1}")
  "P_{xd1, k-1}"/1 -> "P_{d12, k} subsystem"/1("P_{xd1, k-1}"), "P_{xd2, k-1} subsystem"/4("P_{xd1, k-1}")  "P_{xd1, k-1}"

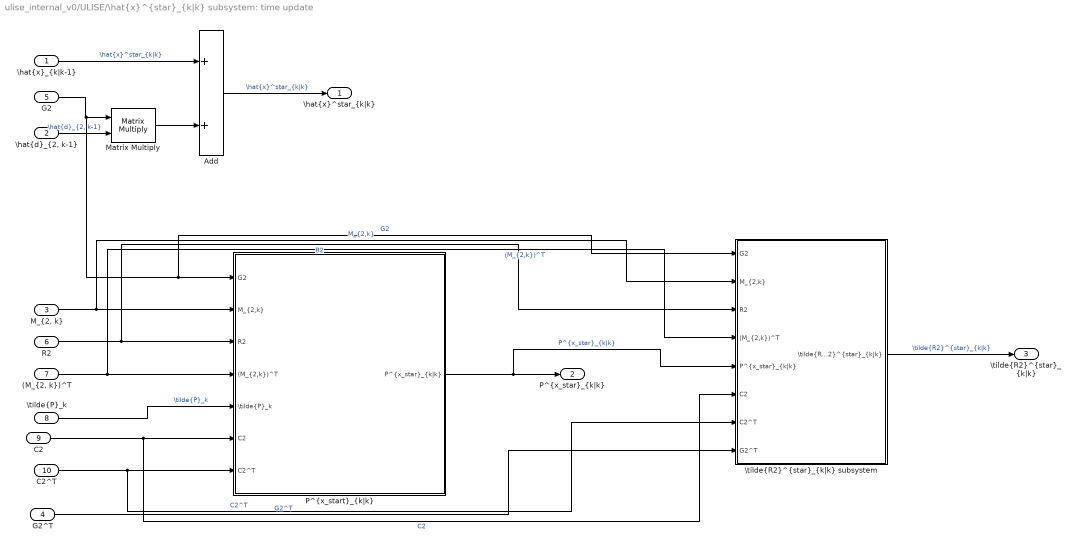
== system ulise_internal_v0/ULISE/\hat{x}^{star}_{k|k} subsystem: time update ==
  "\\hat{x}_{k|k-1}" : Inport
  "\\hat{d}_{2, k-1}" : Inport  Port=2
  "M_{2, k}" : Inport  Port=3
  G2^T : Inport  Port=4
  G2 : Inport  Port=5
  R2 : Inport  Port=6
  "(M_{2, k})^T" : Inport  Port=7
  "\\tilde{P}_k" : Inport  Port=8
  C2 : Inport  Port=9
  C2^T : Inport  Port=10
  Add : Sum
  Matrix Multiply : Product  Multiplication=Matrix(*)
  "P^{x_start}_{k|k}" : Subsystem
  "\\tilde{R2}^{star}_{k|k} subsystem" : Subsystem
  "\\hat{x}^star_{k|k}" : Outport
  "P^{x_star}_{k|k}" : Outport  Port=2
  "\\tilde{R2}^{star}_{k|k}" : Outport  Port=3
  wires:
  "\\hat{d}_{2, k-1}"/1 -> Matrix Multiply/2  "\\hat{d}_{2, k-1}"
  G2/1 -> "\\tilde{R2}^{star}_{k|k} subsystem"/1(G2), "P^{x_start}_{k|k}"/1(G2), Matrix Multiply/1  "G2"
  Matrix Multiply/1 -> Add/2
  "\\hat{x}_{k|k-1}"/1 -> Add/1  "\\hat{x}^star_{k|k}"
  Add/1 -> "\\hat{x}^star_{k|k}"/1  "\\hat{x}^star_{k|k}"
  "M_{2, k}"/1 -> "\\tilde{R2}^{star}_{k|k} subsystem"/2("M_{2,k}"), "P^{x_start}_{k|k}"/2("M_{2,k}")  "M_{2,k}"
  R2/1 -> "\\tilde{R2}^{star}_{k|k} subsystem"/3(R2), "P^{x_start}_{k|k}"/3(R2)  "R2"
  "(M_{2, k})^T"/1 -> "\\tilde{R2}^{star}_{k|k} subsystem"/4("(M_{2,k})^T"), "P^{x_start}_{k|k}"/4("(M_{2,k})^T")  "(M_{2,k})^T"
  "\\tilde{P}_k"/1 -> "P^{x_start}_{k|k}"/5("\\tilde{P}_k")  "\\tilde{P}_k"
  C2/1 -> "\\tilde{R2}^{star}_{k|k} subsystem"/6(C2), "P^{x_start}_{k|k}"/6(C2)  "C2"
  C2^T/1 -> "\\tilde{R2}^{star}_{k|k} subsystem"/7(C2^T), "P^{x_start}_{k|k}"/7(C2^T)  "C2^T"
  "P^{x_start}_{k|k}"/1("P^{x_star}_{k|k}") -> "\\tilde{R2}^{star}_{k|k} subsystem"/5("P^{x_star}_{k|k}"), "P^{x_star}_{k|k}"/1  "P^{x_star}_{k|k}"
  G2^T/1 -> "\\tilde{R2}^{star}_{k|k} subsystem"/8(G2^T)  "G2^T"
  "\\tilde{R2}^{star}_{k|k} subsystem"/1("\\tilde{R2}^{star}_{k|k}") -> "\\tilde{R2}^{star}_{k|k}"/1  "\\tilde{R2}^{star}_{k|k}"

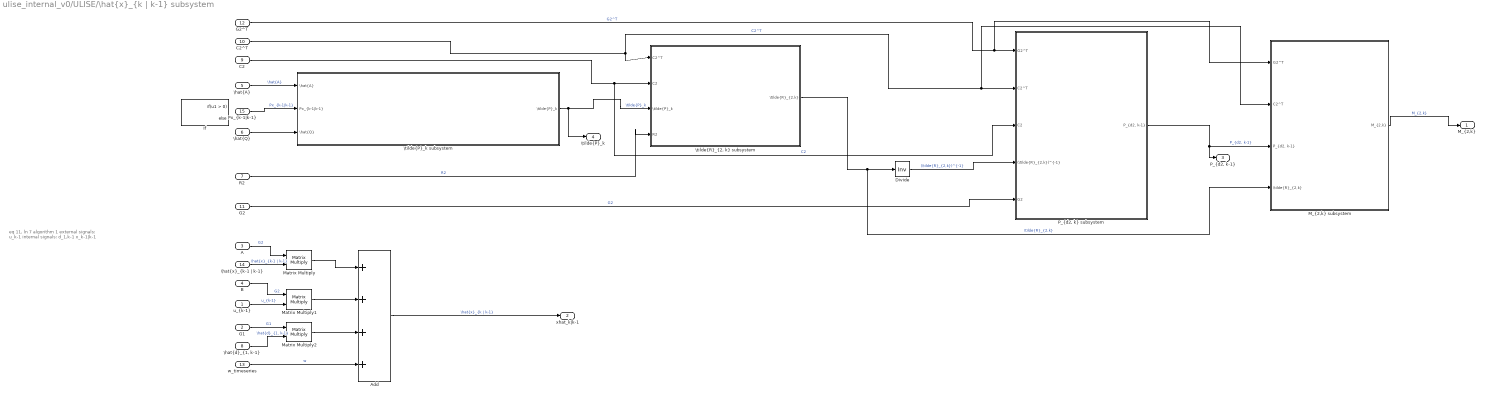
== system ulise_internal_v0/ULISE/\hat{x}_{k | k-1} subsystem ==
  note: eq 11, ln 7 algorithm 1
      | 	external signals:
      | 		u_k-1
      | 	internal signals:
      | 		d_1,k-1
      | 		x_k-1|k-1
  "u_{k-1}" : Inport
  G1 : Inport  Port=2
  A : Inport  Port=3
  B : Inport  Port=4
  "\\hat{A}" : Inport  Port=5
  "\\hat{Q}" : Inport  Port=6
  R2 : Inport  Port=7
  "\\hat{d}_{1, k-1}" : Inport  Port=8
  C2 : Inport  Port=9
  C2^T : Inport  Port=10
  G2 : Inport  Port=11
  G2^T : Inport  Port=12
  w_timeseries : Inport  Port=13
  "\\hat{x}_{k-1 | k-1}" : Inport  Port=14
  "Px_{k-1|k-1}" : Inport  Port=15
  Add : Sum  Inputs=++++
  Divide : Product  Inputs=/  Multiplication=Matrix(*)
  If : If  NumInputs=2
  "M_{2,k} subsystem" : Subsystem
  Matrix Multiply : Product  Multiplication=Matrix(*)
  Matrix Multiply1 : Product  Multiplication=Matrix(*)
  Matrix Multiply2 : Product  Multiplication=Matrix(*)
  "P_{d2, k} subsystem" : Subsystem
  "\\tilde{P}_k subsystem" : Subsystem
  "\\tilde{R}_{2, k} subsystem" : Subsystem
  "M_{2,k}" : Outport
  xhat_k|k-1 : Outport  Port=2
  "P_{d2, k-1}" : Outport  Port=3
  "\\tilde{P}_k" : Outport  Port=4
  wires:
  "\\hat{d}_{1, k-1}"/1 -> Matrix Multiply2/2  "\\hat{d}_{1, k-1}"
  "\\hat{A}"/1 -> "\\tilde{P}_k subsystem"/1("\\hat{A}")  "\\hat{A}"
  "Px_{k-1|k-1}"/1 -> "\\tilde{P}_k subsystem"/2("Px_{k-1|k-1}")  "Px_{k-1|k-1}"
  C2/1 -> "P_{d2, k} subsystem"/3(C2), "\\tilde{R}_{2, k} subsystem"/2(C2)  "C2"
  "\\hat{Q}"/1 -> "\\tilde{P}_k subsystem"/3("\\hat{Q}")
  "\\tilde{P}_k subsystem"/1("\\tilde{P}_k") -> "\\tilde{R}_{2, k} subsystem"/3("\\tilde{P}_k"), "\\tilde{P}_k"/1  "\\tilde{P}_k"
  R2/1 -> "\\tilde{R}_{2, k} subsystem"/4(R2)  "R2"
  C2^T/1 -> "M_{2,k} subsystem"/2(C2^T), "P_{d2, k} subsystem"/2(C2^T), "\\tilde{R}_{2, k} subsystem"/1(C2^T)  "C2^T"
  G2^T/1 -> "M_{2,k} subsystem"/1(G2^T), "P_{d2, k} subsystem"/1(G2^T)  "G2^T"
  G2/1 -> "P_{d2, k} subsystem"/5(G2)  "G2"
  Divide/1 -> "P_{d2, k} subsystem"/4("(\\tilde{R}_{2,k})^{-1}")  "(\\tilde{R}_{2,k})^{-1}"
  "\\tilde{R}_{2, k} subsystem"/1("\\tilde{R}_{2,k}") -> "M_{2,k} subsystem"/4("\\tilde{R}_{2,k}"), Divide/1  "\\tilde{R}_{2,k}"
  "P_{d2, k} subsystem"/1("P_{d2, k-1}") -> "P_{d2, k-1}"/1, "M_{2,k} subsystem"/3("P_{d2, k-1}")  "P_{d2, k-1}"
  "M_{2,k} subsystem"/1("M_{2,k}") -> "M_{2,k}"/1  "M_{2,k}"
  Matrix Multiply/1 -> Add/1
  Matrix Multiply1/1 -> Add/2
  Matrix Multiply2/1 -> Add/3
  B/1 -> Matrix Multiply1/1  "G2"
  G1/1 -> Matrix Multiply2/1  "G1"
  w_timeseries/1 -> Add/4  "w"
  Add/1 -> xhat_k|k-1/1  "\\hat{x}_{k | k-1}"
  "u_{k-1}"/1 -> Matrix Multiply1/2  "u_{k-1}"
  A/1 -> Matrix Multiply/1  "G2"
  "\\hat{x}_{k-1 | k-1}"/1 -> Matrix Multiply/2  "\\hat{x}_{k-1 | k-1}"

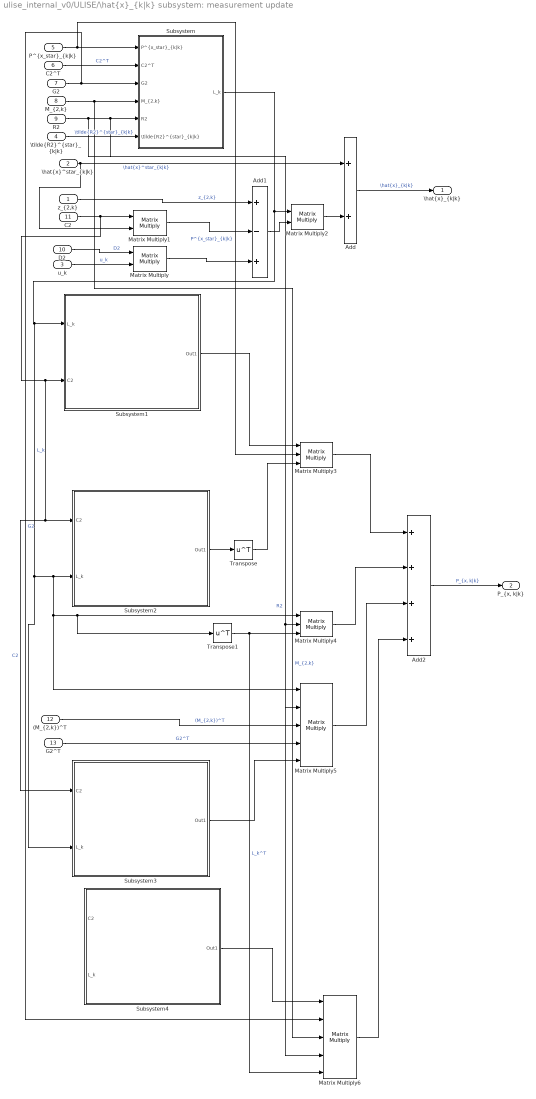
== system ulise_internal_v0/ULISE/\hat{x}_{k|k} subsystem: measurement update ==
  "z_{2,k}" : Inport
  "\\hat{x}^star_{k|k}" : Inport  Port=2
  u_k : Inport  Port=3
  "\\tilde{R2}^{star}_{k|k}" : Inport  Port=4
  "P^{x_star}_{k|k}" : Inport  Port=5
  C2^T : Inport  Port=6
  G2 : Inport  Port=7
  "M_{2,k}" : Inport  Port=8
  R2 : Inport  Port=9
  D2 : Inport  Port=10
  C2 : Inport  Port=11
  "(M_{2,k})^T" : Inport  Port=12
  G2^T : Inport  Port=13
  Add : Sum
  Add1 : Sum  Inputs=+-+
  Add2 : Sum  Inputs=++++
  Matrix Multiply : Product  Multiplication=Matrix(*)
  Matrix Multiply1 : Product  Multiplication=Matrix(*)
  Matrix Multiply2 : Product  Multiplication=Matrix(*)
  Matrix Multiply3 : Product  Inputs=3  Multiplication=Matrix(*)
  Matrix Multiply4 : Product  Inputs=3  Multiplication=Matrix(*)
  Matrix Multiply5 : Product  Inputs=5  Multiplication=Matrix(*)
  Matrix Multiply6 : Product  Inputs=5  Multiplication=Matrix(*)
  Subsystem : Subsystem
  Subsystem1 : Subsystem
  Subsystem2 : Subsystem
  Subsystem3 : Subsystem
  Subsystem4 : Subsystem
  Transpose : Math  Operator=transpose
  Transpose1 : Math  Operator=transpose
  "\\hat{x}_{k|k}" : Outport
  "P_{x, k|k}" : Outport  Port=2
  wires:
  "P^{x_star}_{k|k}"/1 -> Matrix Multiply3/2, Subsystem/1("P^{x_star}_{k|k}")  "P^{x_star}_{k|k}"
  C2^T/1 -> Subsystem/2(C2^T)  "C2^T"
  G2/1 -> Matrix Multiply6/2, Subsystem/3(G2)  "G2"
  "M_{2,k}"/1 -> Matrix Multiply6/3, Subsystem/4("M_{2,k}")  "M_{2,k}"
  R2/1 -> Matrix Multiply6/4, Matrix Multiply5/2, Matrix Multiply4/2, Subsystem/5(R2)  "R2"
  "\\tilde{R2}^{star}_{k|k}"/1 -> Subsystem/6("\\tilde{R2}^{star}_{k|k}")  "\\tilde{R2}^{star}_{k|k}"
  Subsystem/1(L_k) -> Subsystem3/2(L_k), Matrix Multiply5/1, Transpose1/1, Matrix Multiply4/1, Subsystem2/2(L_k), Subsystem1/1(L_k), Matrix Multiply2/1  "L_k"
  Add/1 -> "\\hat{x}_{k|k}"/1  "\\hat{x}_{k|k}"
  "\\hat{x}^star_{k|k}"/1 -> Add/1, Matrix Multiply1/2  "\\hat{x}^star_{k|k}"
  D2/1 -> Matrix Multiply/1  "D2"
  "z_{2,k}"/1 -> Add1/1  "z_{2,k}"
  u_k/1 -> Matrix Multiply/2  "u_k"
  Matrix Multiply/1 -> Add1/3
  C2/1 -> Subsystem2/1(C2), Subsystem3/1(C2), Subsystem1/2(C2), Matrix Multiply1/1  "C2"
  Matrix Multiply1/1 -> Add1/2
  Add1/1 -> Matrix Multiply2/2
  Matrix Multiply2/1 -> Add/2
  Subsystem1/1(Out1) -> Matrix Multiply3/1
  Subsystem2/1(Out1) -> Transpose/1
  Transpose/1 -> Matrix Multiply3/3
  Matrix Multiply3/1 -> Add2/1
  Matrix Multiply4/1 -> Add2/2
  Transpose1/1 -> Matrix Multiply6/5, Matrix Multiply4/3  "L_k^T"
  Matrix Multiply5/1 -> Add2/3
  "(M_{2,k})^T"/1 -> Matrix Multiply5/3  "(M_{2,k})^T"
  G2^T/1 -> Matrix Multiply5/4  "G2^T"
  Subsystem3/1(Out1) -> Matrix Multiply5/5
  Matrix Multiply6/1 -> Add2/4
  Subsystem4/1(Out1) -> Matrix Multiply6/1
  Add2/1 -> "P_{x, k|k}"/1  "P_{x, k|k}"

== system ulise_internal_v0/ULISE/\hat{d}_{1, k} subsystem/P_{xd1, k} subsystem ==
  "P_{x, k|k}" : Inport
  C1^T : Inport  Port=2
  M1^T : Inport  Port=3
  Add1 : Sum  Inputs=-
  Matrix Multiply2 : Product  Inputs=3  Multiplication=Matrix(*)
  "P_{xd1, k}" : Outport
  wires:
  "P_{x, k|k}"/1 -> Add1/1
  Matrix Multiply2/1 -> "P_{xd1, k}"/1  "P_{xd1, k}"
  M1^T/1 -> Matrix Multiply2/3
  C1^T/1 -> Matrix Multiply2/2
  Add1/1 -> Matrix Multiply2/1  "-P_{x, k|k}"

== system ulise_internal_v0/ULISE/\hat{d}_{1, k} subsystem/Subsystem ==
  R1 : Inport
  "P_{x, k|k}" : Inport  Port=2
  C1^T : Inport  Port=3
  M1 : Inport  Port=4
  C1 : Inport  Port=5
  Add1 : Sum
  Matrix Multiply3 : Product  Inputs=3  Multiplication=Matrix(*)
  Matrix Multiply4 : Product  Inputs=3  Multiplication=Matrix(*)
  "P_{d1, k|k}" : Outport
  wires:
  Matrix Multiply4/1 -> "P_{d1, k|k}"/1  "P_{d1, k|k}"
  C1/1 -> Matrix Multiply3/1
  M1/1 -> Matrix Multiply4/1, Matrix Multiply4/3
  C1^T/1 -> Matrix Multiply3/3
  "P_{x, k|k}"/1 -> Matrix Multiply3/2
  Matrix Multiply3/1 -> Add1/2
  R1/1 -> Add1/1
  Add1/1 -> Matrix Multiply4/2  "\\tilde{R1}_{k|k}"

== system ulise_internal_v0/ULISE/\hat{d}_{1, k} subsystem/Subsystem1 ==
  V1^T : Inport
  V2^T : Inport  Port=2
  "P_{xd1, k-1}" : Inport  Port=3
  "P_{xd2, k-1}" : Inport  Port=4
  Add3 : Sum
  Matrix Multiply10 : Product  Multiplication=Matrix(*)
  Matrix Multiply8 : Product  Multiplication=Matrix(*)
  "P_{xd, k-1}" : Outport
  wires:
  V1^T/1 -> Matrix Multiply8/2  "V1^T"
  "P_{xd1, k-1}"/1 -> Matrix Multiply8/1  "P_{xd1, k-1}"
  Matrix Multiply10/1 -> Add3/2  "P_[xd2, k-1}*V2^T"
  Matrix Multiply8/1 -> Add3/1  "P_{xd1, k-1}*V1^T"
  V2^T/1 -> Matrix Multiply10/2  "V2^T"
  Add3/1 -> "P_{xd, k-1}"/1  "P_{xd, k-1}"
  "P_{xd2, k-1}"/1 -> Matrix Multiply10/1  "P_{xd2, k-1}"

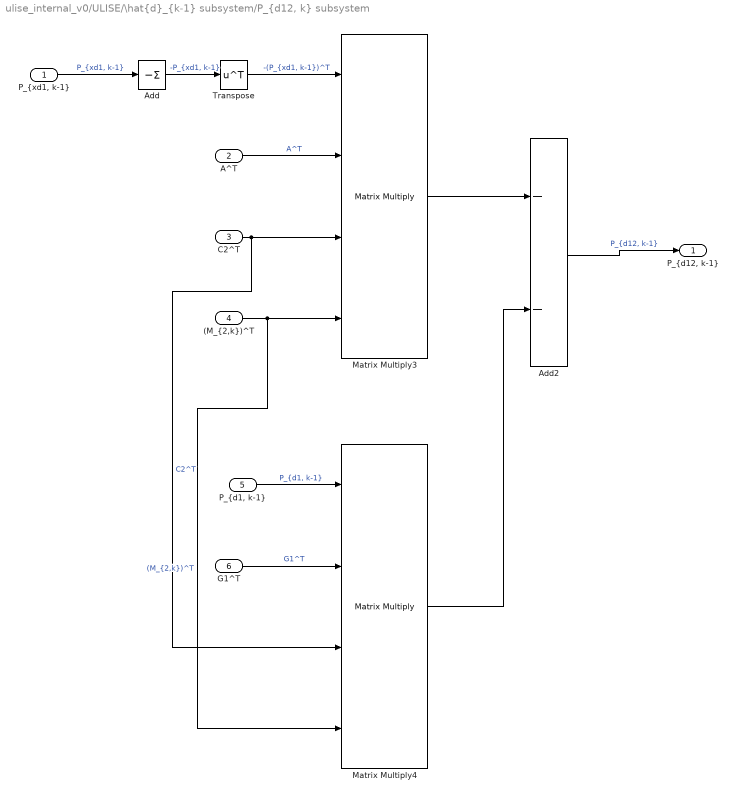
== system ulise_internal_v0/ULISE/\hat{d}_{k-1} subsystem/P_{d12, k} subsystem ==
  "P_{xd1, k-1}" : Inport
  A^T : Inport  Port=2
  C2^T : Inport  Port=3
  "(M_{2,k})^T" : Inport  Port=4
  "P_{d1, k-1}" : Inport  Port=5
  G1^T : Inport  Port=6
  Add : Sum  Inputs=-
  Add2 : Sum  Inputs=--
  Matrix Multiply3 : Product  Inputs=4  Multiplication=Matrix(*)
  Matrix Multiply4 : Product  Inputs=4  Multiplication=Matrix(*)
  Transpose : Math  Operator=transpose
  "P_{d12, k-1}" : Outport
  wires:
  "P_{xd1, k-1}"/1 -> Add/1  "P_{xd1, k-1}"
  Add2/1 -> "P_{d12, k-1}"/1  "P_{d12, k-1}"
  "P_{d1, k-1}"/1 -> Matrix Multiply4/1  "P_{d1, k-1}"
  Transpose/1 -> Matrix Multiply3/1  "-(P_{xd1, k-1})^T"
  G1^T/1 -> Matrix Multiply4/2  "G1^T"
  Matrix Multiply3/1 -> Add2/1
  C2^T/1 -> Matrix Multiply3/3, Matrix Multiply4/3  "C2^T"
  "(M_{2,k})^T"/1 -> Matrix Multiply3/4, Matrix Multiply4/4  "(M_{2,k})^T"
  Matrix Multiply4/1 -> Add2/2
  A^T/1 -> Matrix Multiply3/2  "A^T"
  Add/1 -> Transpose/1  "-P_{xd1, k-1}"

== system ulise_internal_v0/ULISE/\hat{d}_{k-1} subsystem/P_{xd2, k-1} subsystem ==
  "Px_{k-1|k-1}" : Inport
  A^T : Inport  Port=2
  C2^T : Inport  Port=3
  "P_{xd1, k-1}" : Inport  Port=4
  "(M_{2,k})^T" : Inport  Port=5
  Add2 : Sum  Inputs=--
  Matrix Multiply5 : Product  Inputs=4  Multiplication=Matrix(*)
  Matrix Multiply6 : Product  Inputs=4  Multiplication=Matrix(*)
  "P_{xd2, k-1}" : Outport
  wires:
  "Px_{k-1|k-1}"/1 -> Matrix Multiply5/1  "Px_{k-1|k-1}"
  Matrix Multiply5/1 -> Add2/1
  "P_{xd1, k-1}"/1 -> Matrix Multiply6/1  "P_{xd1, k-1}"
  C2^T/1 -> Matrix Multiply5/3, Matrix Multiply6/3  "C2^T"
  Add2/1 -> "P_{xd2, k-1}"/1  "P_{xd2, k-1}"
  "(M_{2,k})^T"/1 -> Matrix Multiply6/4, Matrix Multiply5/4  "(M_{2,k})^T"
  Matrix Multiply6/1 -> Add2/2
  A^T/1 -> Matrix Multiply5/2, Matrix Multiply6/2  "A^T"

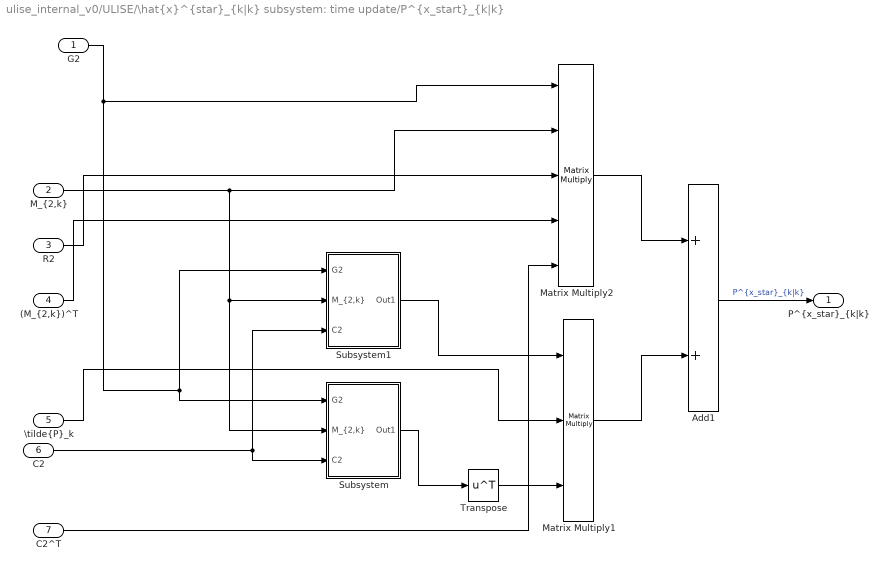
== system ulise_internal_v0/ULISE/\hat{x}^{star}_{k|k} subsystem: time update/P^{x_start}_{k|k} ==
  G2 : Inport
  "M_{2,k}" : Inport  Port=2
  R2 : Inport  Port=3
  "(M_{2,k})^T" : Inport  Port=4
  "\\tilde{P}_k" : Inport  Port=5
  C2 : Inport  Port=6
  C2^T : Inport  Port=7
  Add1 : Sum
  Matrix Multiply1 : Product  Inputs=3  Multiplication=Matrix(*)
  Matrix Multiply2 : Product  Inputs=5  Multiplication=Matrix(*)
  Subsystem : Subsystem
  Subsystem1 : Subsystem
  Transpose : Math  Operator=transpose
  "P^{x_star}_{k|k}" : Outport
  wires:
  R2/1 -> Matrix Multiply2/3
  Subsystem1/1(Out1) -> Matrix Multiply1/1
  Add1/1 -> "P^{x_star}_{k|k}"/1  "P^{x_star}_{k|k}"
  Transpose/1 -> Matrix Multiply1/3
  Matrix Multiply1/1 -> Add1/2
  Matrix Multiply2/1 -> Add1/1
  C2^T/1 -> Matrix Multiply2/5
  "(M_{2,k})^T"/1 -> Matrix Multiply2/4
  "\\tilde{P}_k"/1 -> Matrix Multiply1/2
  G2/1 -> Matrix Multiply2/1, Subsystem1/1(G2), Subsystem/1(G2)
  Subsystem/1(Out1) -> Transpose/1
  C2/1 -> Subsystem1/3(C2), Subsystem/3(C2)
  "M_{2,k}"/1 -> Matrix Multiply2/2, Subsystem/2("M_{2,k}"), Subsystem1/2("M_{2,k}")

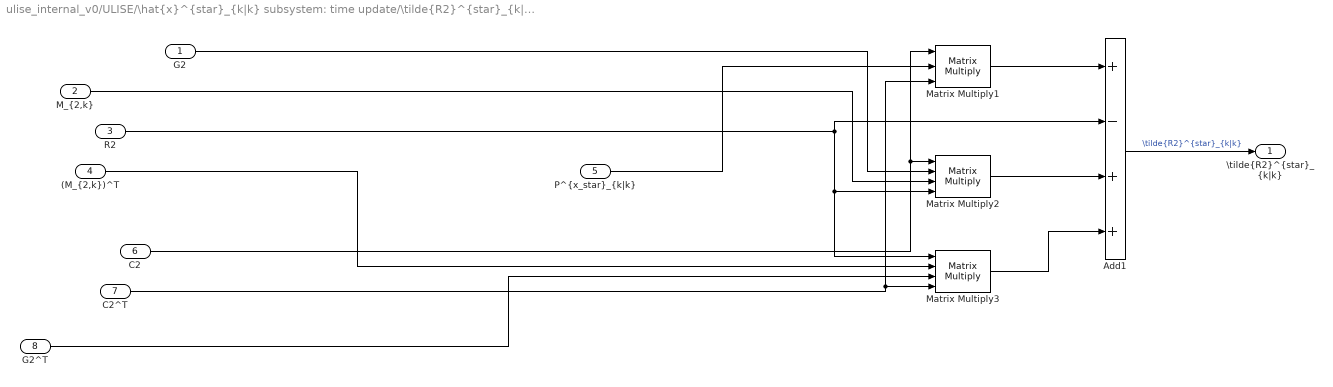
== system ulise_internal_v0/ULISE/\hat{x}^{star}_{k|k} subsystem: time update/\tilde{R2}^{star}_{k|k} subsystem ==
  G2 : Inport
  "M_{2,k}" : Inport  Port=2
  R2 : Inport  Port=3
  "(M_{2,k})^T" : Inport  Port=4
  "P^{x_star}_{k|k}" : Inport  Port=5
  C2 : Inport  Port=6
  C2^T : Inport  Port=7
  G2^T : Inport  Port=8
  Add1 : Sum  Inputs=+-++
  Matrix Multiply1 : Product  Inputs=3  Multiplication=Matrix(*)
  Matrix Multiply2 : Product  Inputs=4  Multiplication=Matrix(*)
  Matrix Multiply3 : Product  Inputs=4  Multiplication=Matrix(*)
  "\\tilde{R2}^{star}_{k|k}" : Outport
  wires:
  Add1/1 -> "\\tilde{R2}^{star}_{k|k}"/1  "\\tilde{R2}^{star}_{k|k}"
  Matrix Multiply3/1 -> Add1/4
  "P^{x_star}_{k|k}"/1 -> Matrix Multiply1/2
  C2^T/1 -> Matrix Multiply1/3, Matrix Multiply3/4
  C2/1 -> Matrix Multiply2/1, Matrix Multiply1/1
  R2/1 -> Add1/2, Matrix Multiply3/1, Matrix Multiply2/4
  G2/1 -> Matrix Multiply2/2
  G2^T/1 -> Matrix Multiply3/3
  "M_{2,k}"/1 -> Matrix Multiply2/3
  "(M_{2,k})^T"/1 -> Matrix Multiply3/2
  Matrix Multiply2/1 -> Add1/3
  Matrix Multiply1/1 -> Add1/1

== system ulise_internal_v0/ULISE/\hat{x}_{k | k-1} subsystem/M_{2,k} subsystem ==
  G2^T : Inport
  C2^T : Inport  Port=2
  "P_{d2, k-1}" : Inport  Port=3
  "\\tilde{R}_{2,k}" : Inport  Port=4
  Matrix Multiply : Product  Inputs=4  Multiplication=Matrix(*)
  "M_{2,k}" : Outport
  wires:
  "\\tilde{R}_{2,k}"/1 -> Matrix Multiply/4
  C2^T/1 -> Matrix Multiply/3
  G2^T/1 -> Matrix Multiply/2
  "P_{d2, k-1}"/1 -> Matrix Multiply/1  "P_{d2, k-1}"
  Matrix Multiply/1 -> "M_{2,k}"/1  "M_{2,k}"

== system ulise_internal_v0/ULISE/\hat{x}_{k | k-1} subsystem/P_{d2, k} subsystem ==
  G2^T : Inport
  C2^T : Inport  Port=2
  C2 : Inport  Port=3
  "(\\tilde{R}_{2,k})^{-1}" : Inport  Port=4
  G2 : Inport  Port=5
  Divide : Product  Inputs=/  Multiplication=Matrix(*)
  Matrix Multiply1 : Product  Inputs=5  Multiplication=Matrix(*)
  "P_{d2, k-1}" : Outport
  wires:
  G2^T/1 -> Matrix Multiply1/1  "G2^T"
  G2/1 -> Matrix Multiply1/5  "G2"
  "(\\tilde{R}_{2,k})^{-1}"/1 -> Matrix Multiply1/3  "{\\tilde{R}_{2, k})^{-1}"
  Divide/1 -> "P_{d2, k-1}"/1  "P_{d2, k}"
  C2/1 -> Matrix Multiply1/4  "C2"
  C2^T/1 -> Matrix Multiply1/2  "C2^T"
  Matrix Multiply1/1 -> Divide/1

== system ulise_internal_v0/ULISE/\hat{x}_{k | k-1} subsystem/\tilde{P}_k subsystem ==
  "\\hat{A}" : Inport
  "Px_{k-1|k-1}" : Inport  Port=2
  "\\hat{Q}" : Inport  Port=3
  Add : Sum
  Matrix Multiply : Product  Inputs=3  Multiplication=Matrix(*)
  Transpose : Math  Operator=transpose  OutputSignalType=real
  "\\tilde{P}_k" : Outport
  wires:
  Add/1 -> "\\tilde{P}_k"/1  "\\tilde{P}_k"
  Transpose/1 -> Matrix Multiply/3  "\\hat{A}^T"
  "Px_{k-1|k-1}"/1 -> Matrix Multiply/2  "P_{k-1 | k-1}"
  Matrix Multiply/1 -> Add/1
  "\\hat{Q}"/1 -> Add/2  "\\hat{Q}"
  "\\hat{A}"/1 -> Matrix Multiply/1, Transpose/1

== system ulise_internal_v0/ULISE/\hat{x}_{k | k-1} subsystem/\tilde{R}_{2, k} subsystem ==
  note: \tilde{R}_{2, k} subsystem
  C2^T : Inport
  C2 : Inport  Port=2
  "\\tilde{P}_k" : Inport  Port=3
  R2 : Inport  Port=4
  Add : Sum
  Matrix Multiply1 : Product  Inputs=3  Multiplication=Matrix(*)
  "\\tilde{R}_{2,k}" : Outport
  wires:
  Matrix Multiply1/1 -> Add/1
  C2/1 -> Matrix Multiply1/1
  Add/1 -> "\\tilde{R}_{2,k}"/1  "\\tilde{R}_{2,k}"
  R2/1 -> Add/2
  C2^T/1 -> Matrix Multiply1/3
  "\\tilde{P}_k"/1 -> Matrix Multiply1/2

== system ulise_internal_v0/ULISE/\hat{x}_{k|k} subsystem: measurement update/Subsystem ==
  "P^{x_star}_{k|k}" : Inport
  C2^T : Inport  Port=2
  G2 : Inport  Port=3
  "M_{2,k}" : Inport  Port=4
  R2 : Inport  Port=5
  "\\tilde{R2}^{star}_{k|k}" : Inport  Port=6
  Add : Sum
  Matrix Multiply : Product  Multiplication=Matrix(*)
  Matrix Multiply1 : Product  Inputs=3  Multiplication=Matrix(*)
  Matrix Multiply2 : Product  Multiplication=Matrix(*)
  L_k : Outport
  wires:
  C2^T/1 -> Matrix Multiply/2
  "P^{x_star}_{k|k}"/1 -> Matrix Multiply/1
  Matrix Multiply2/1 -> L_k/1  "L_k"
  "M_{2,k}"/1 -> Matrix Multiply1/2
  G2/1 -> Matrix Multiply1/1
  Add/1 -> Matrix Multiply2/1
  "\\tilde{R2}^{star}_{k|k}"/1 -> Matrix Multiply2/2
  R2/1 -> Matrix Multiply1/3
  Matrix Multiply/1 -> Add/1
  Matrix Multiply1/1 -> Add/2

== system ulise_internal_v0/ULISE/\hat{x}_{k|k} subsystem: measurement update/Subsystem1 ==
  L_k : Inport
  C2 : Inport  Port=2
  Add2 : Sum  Inputs=+-
  Constant : Constant  Value=eye(size(x,1))
  Matrix Multiply3 : Product  Multiplication=Matrix(*)
  Out1 : Outport
  wires:
  Add2/1 -> Out1/1
  Constant/1 -> Add2/1  "I_nxn"
  C2/1 -> Matrix Multiply3/2
  L_k/1 -> Matrix Multiply3/1
  Matrix Multiply3/1 -> Add2/2

== system ulise_internal_v0/ULISE/\hat{x}_{k|k} subsystem: measurement update/Subsystem2 ==
  C2 : Inport
  L_k : Inport  Port=2
  Add2 : Sum  Inputs=+-
  Constant : Constant  Value=eye(size(x,1))
  Matrix Multiply3 : Product  Multiplication=Matrix(*)
  Out1 : Outport
  wires:
  Add2/1 -> Out1/1
  Constant/1 -> Add2/1  "I_nxn"
  C2/1 -> Matrix Multiply3/2
  L_k/1 -> Matrix Multiply3/1
  Matrix Multiply3/1 -> Add2/2

== system ulise_internal_v0/ULISE/\hat{x}_{k|k} subsystem: measurement update/Subsystem3 ==
  C2 : Inport
  L_k : Inport  Port=2
  Add2 : Sum  Inputs=+-
  Constant : Constant  Value=eye(size(x,1))
  Matrix Multiply3 : Product  Multiplication=Matrix(*)
  Out1 : Outport
  wires:
  Add2/1 -> Out1/1
  Constant/1 -> Add2/1  "I_nxn"
  C2/1 -> Matrix Multiply3/2
  L_k/1 -> Matrix Multiply3/1
  Matrix Multiply3/1 -> Add2/2

== system ulise_internal_v0/ULISE/\hat{x}_{k|k} subsystem: measurement update/Subsystem4 ==
  C2 : Inport
  L_k : Inport  Port=2
  Add2 : Sum  Inputs=+-
  Constant : Constant  Value=eye(size(x,1))
  Matrix Multiply3 : Product  Multiplication=Matrix(*)
  Out1 : Outport
  wires:
  Add2/1 -> Out1/1
  Constant/1 -> Add2/1  "I_nxn"
  C2/1 -> Matrix Multiply3/2
  L_k/1 -> Matrix Multiply3/1
  Matrix Multiply3/1 -> Add2/2

== system ulise_internal_v0/ULISE/\hat{x}^{star}_{k|k} subsystem: time update/P^{x_start}_{k|k}/Subsystem ==
  G2 : Inport
  "M_{2,k}" : Inport  Port=2
  C2 : Inport  Port=3
  Add1 : Sum
  Constant : Constant  Value=eye(size(x,1))
  Matrix Multiply1 : Product  Inputs=3  Multiplication=Matrix(*)
  Out1 : Outport
  wires:
  G2/1 -> Matrix Multiply1/1
  C2/1 -> Matrix Multiply1/3
  Add1/1 -> Out1/1
  Matrix Multiply1/1 -> Add1/2
  "M_{2,k}"/1 -> Matrix Multiply1/2
  Constant/1 -> Add1/1  "I_nxn"

== system ulise_internal_v0/ULISE/\hat{x}^{star}_{k|k} subsystem: time update/P^{x_start}_{k|k}/Subsystem1 ==
  G2 : Inport
  "M_{2,k}" : Inport  Port=2
  C2 : Inport  Port=3
  Add1 : Sum
  Constant : Constant  Value=eye(size(x,1))
  Matrix Multiply1 : Product  Inputs=3  Multiplication=Matrix(*)
  Out1 : Outport
  wires:
  G2/1 -> Matrix Multiply1/1
  C2/1 -> Matrix Multiply1/3
  Add1/1 -> Out1/1
  Matrix Multiply1/1 -> Add1/2
  "M_{2,k}"/1 -> Matrix Multiply1/2
  Constant/1 -> Add1/1  "I_nxn"

== matlab function ulise_internal_v0/MATLAB Function ==
  data: x input; x_out output; K input
function x_out = fcn(x,K)

persistent k 

% Initialize x_out
x_out = zeros( size(x,1), K );

% Update 
x_out(:, k) = x;

% Time update 
k = k + 1;

== matlab function ulise_internal_v0/ULISE/MATLAB Function ==
  data: H input; U1 output; U2 output; S output; V1 output; V2 output
function [U1,U2, S, V1, V2] = full_svd(H)
 
% Define the rank of H
r = rank(H);

% Singular Value Decomposition of H
[U, S, V] = svd(H);
%
U1 = U(:,1:r);
U2 = U(:,r+1:end);
%
S = S(1:r,1:r);
%
V1 = V(:,1:r);
V2 = V(:,r+1:end);
